simulink library "rw_motor_lib_disc"  (R2018b)
settings: Solver=VariableStepAuto  StartTime=0.0  StopTime=10.0  RelTol=1e-3
undefined symbols (not defined in the file): simParams
libraries: simulink x1
settings Model: Creator=Taylor  LastModifiedBy=taylorreynolds

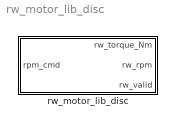
== system rw_motor_lib_disc ==
  rw_motor_lib_disc : Subsystem  mask{id_a=1}
      mask prompts: id_a "Choose the actuator ID."
      mask TypeOptions id_a: 1 | 2 | 3 | 4
      mask DialogControl DescTextVar Prompt: SOCi reaction wheel model

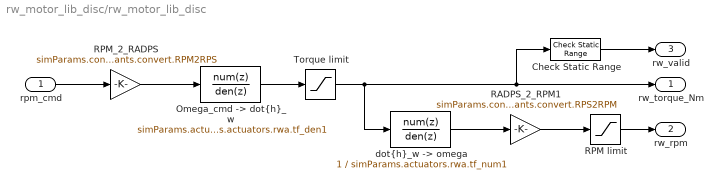
== system rw_motor_lib_disc/rw_motor_lib_disc ==
  rpm_cmd : Inport
  Check Static Range : simulink/Model Verification/Check  Static Range  Description=-simParams.actuators.rwa.max_torque_Nm < u < simParams.actuators.rwa.max_torque_Nm  max=simParams.actuators.rwa.max_torque_Nm  max_included=off  min=-simParams.actuators.rwa.max_torque_Nm  min_included=off  enabled=on  stopWhenAssertionFail=off  export=on  icon=graphic
      settings: SourceProductName=Simulink  SourceProductBaseCode=SL
  "Omega_cmd -> dot{h}_w" : DiscreteTransferFcn  Numerator=simParams.actuators.rwa.tf_num1  Denominator=simParams.actuators.rwa.tf_den1
  RADPS_2_RPM1 : Gain  Gain=simParams.constants.convert.RPS2RPM
  RPM limit : Saturate  UpperLimit=simParams.actuators.rwa.max_RPM  LowerLimit=-simParams.actuators.rwa.max_RPM
  RPM_2_RADPS : Gain  Gain=simParams.constants.convert.RPM2RPS
  Torque limit : Saturate  UpperLimit=simParams.actuators.rwa.max_torque_Nm  LowerLimit=-simParams.actuators.rwa.max_torque_Nm
  "dot{h}_w -> omega" : DiscreteTransferFcn  Numerator=1  Denominator=simParams.actuators.rwa.tf_num1  InitialStates=simParams.initialConditions.rwa.radps(id_a)
  rw_torque_Nm : Outport
  rw_rpm : Outport  Port=2
  rw_valid : Outport  Port=3
  wires:
  rpm_cmd/1 -> RPM_2_RADPS/1
  RPM_2_RADPS/1 -> "Omega_cmd -> dot{h}_w"/1
  "Omega_cmd -> dot{h}_w"/1 -> Torque limit/1
  Check Static Range/1 -> rw_valid/1
  "dot{h}_w -> omega"/1 -> RADPS_2_RPM1/1
  RADPS_2_RPM1/1 -> RPM limit/1
  Torque limit/1 -> "dot{h}_w -> omega"/1, Check Static Range/1, rw_torque_Nm/1
  RPM limit/1 -> rw_rpm/1
